simulink model "PROJECT_SIMULINK_LINEAR_BICYCLE_VLiam3"  (R2023b)
settings: Solver=ode4  StartTime=0.0  StopTime=20  FixedStep=1e-3  RelTol=1e-3  EnableMultiTasking=on
values from neighbouring files (symbols this model uses):
  Ts = 0.01    [PROJECT_INIT_LINEAR_BICYCLE_VLiam3.m]
  V_ref = 60 /3.6    (= 16.6666666667)    [PROJECT_INIT_LINEAR_BICYCLE_VLiam3.m]    (also in run_template.m)
undefined symbols (not defined in the file or in its folder): data, init, input, par
libraries: simulink x2
settings Model: Creator=bshyrokau  LastModifiedBy=liamr
settings SolverCC: AlgebraicLoopSolver=TrustRegion  AutoInsertRateTranBlk=on
settings DataIOCC: SaveOutput=off  SignalLogging=off  DSMLogging=off  SaveTime=off  ReturnWorkspaceOutputs=off
settings OptimizationCC: ReuseModelBlockBuffer=off  LifeSpan=inf
settings DebuggingCC: UnconnectedInputMsg=warning  UnconnectedOutputMsg=warning  UnconnectedLineMsg=warning  AllowSymbolicDim=off  SFUnexpectedBacktrackingDiag=warning  SFNoUnconditionalDefaultTransitionDiag=warning  SFExecutionAtInitializationDiag=none  ArithmeticOperatorsInVariantConditions=warning
settings ModelReferenceCC: EnableRefExpFcnMdlSchedulingChecks=on  PropagateSignalLabelsOutOfModel=off
settings SFSimCC: SimUseLocalCustomCode=off  CustomCodeUndefinedFunction=UseInterfaceOnly
settings RTWCC: RTWUseLocalCustomCode=off  DLArmComputeVersion=19.05
settings CodeAppCC: StateflowObjectComments=on
settings GRTTargetCC: TargetLangStandard=C89/C90 (ANSI)
settings ConfigComp: CovMetricSettings=dw  CovSaveCumulativeToWorkspaceVar=on  CovSaveSingleToWorkspaceVar=on  CovExternalEMLEnable=off
settings SimscapeCC: SimscapeNormalizeSystem=off
settings ConfigurationSet: Description=SimMechanics 2G

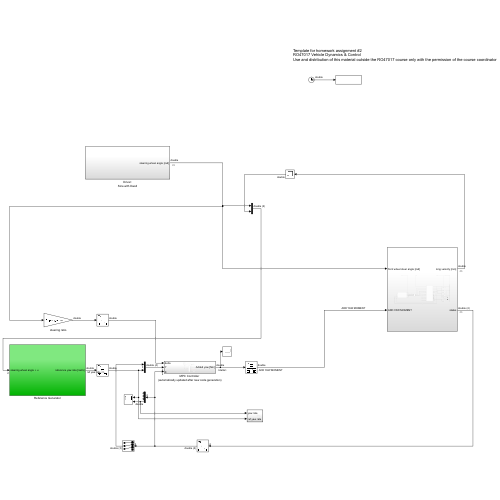
[thumbnail: Simulink's stored preview of the top-level diagram]
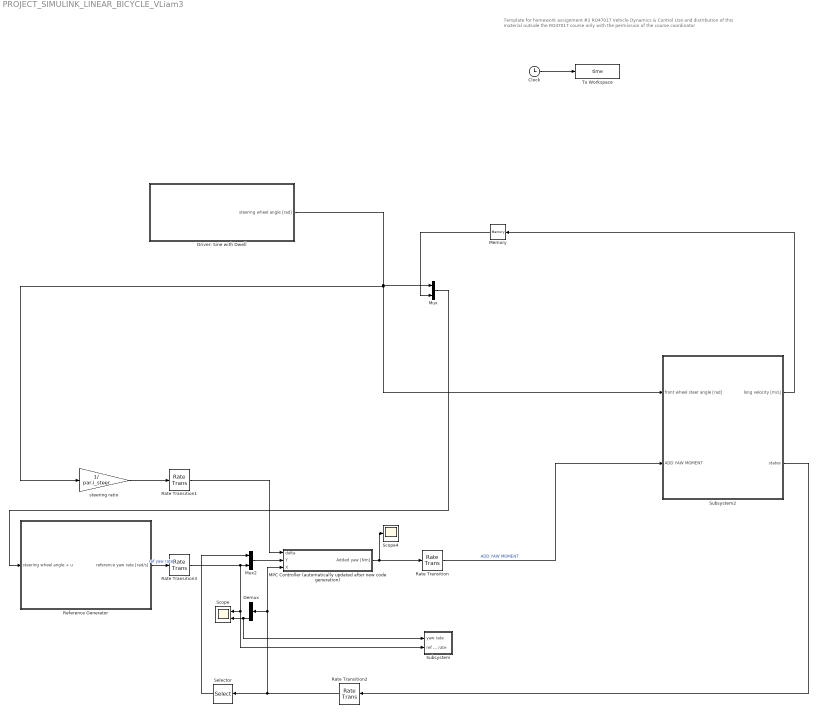
== system PROJECT_SIMULINK_LINEAR_BICYCLE_VLiam3 ==
  note: Template for homework assignment #2
      | RO47017 Vehicle Dynamics & Control
      | Use and distribution of this material outside the RO47017 course only with the permission of the course coordinator
  Clock : Clock
  Demux : Demux
  Driver: Sine with Dwell : Subsystem
  MPC Controller (automatically updated after new code generation) : Subsystem
  Memory : Memory
  Mux : Mux  Inputs=2
  Mux2 : Mux  Inputs=2
  Rate Transition : RateTransition
  Rate Transition1 : RateTransition  OutPortSampleTime=Ts
  Rate Transition2 : RateTransition  OutPortSampleTime=Ts
  Rate Transition3 : RateTransition  OutPortSampleTime=Ts
  Reference Generator : Subsystem  StartFcn=veh_parameters
  Scope : Scope  NumInputPorts=2
  Scope4 : Scope
  Selector : Selector  InputPortWidth=4  IndexOptions=Index vector (dialog)  Indices=[1 2 3]  OutputSizes=1
  Subsystem : Subsystem
  Subsystem2 : Subsystem
  To Workspace : ToWorkspace  VariableName=time  SampleTime=-1
  steering ratio : Gain  Gain=1/ par.i_steer
  wires:
  Driver: Sine with Dwell/1(steering wheel angle [rad]) -> Subsystem2/1(front wheel steer angle [rad]), steering ratio/1, Mux/1
  Clock/1 -> To Workspace/1
  MPC Controller (automatically updated after new code generation)/1(Added yaw [Nm]) -> Scope4/1, Rate Transition/1
  Rate Transition2/1 -> Selector/1, Demux/1, MPC Controller (automatically updated after new code generation)/3(X)
  Mux/1 -> Reference Generator/1(steering wheel angle + u)
  Rate Transition1/1 -> MPC Controller (automatically updated after new code generation)/1(delta)
  Memory/1 -> Mux/2
  Reference Generator/1(reference yaw rate [rad/s]) -> Rate Transition3/1  "ref yaw rate"
  Selector/1 -> Mux2/1
  Rate Transition3/1 -> Subsystem/2(ref yaw rate), Scope/1, Mux2/2
  Mux2/1 -> MPC Controller (automatically updated after new code generation)/2(Y)
  steering ratio/1 -> Rate Transition1/1
  Demux/4 -> Subsystem/1(yaw rate), Scope/2
  Rate Transition/1 -> Subsystem2/2(ADD YAW MOMENT)  "ADD YAW MOMENT"
  Subsystem2/1(long velocity [m/s]) -> Memory/1
  Subsystem2/2(states) -> Rate Transition2/1

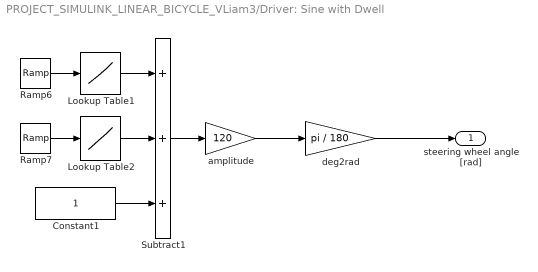
== system PROJECT_SIMULINK_LINEAR_BICYCLE_VLiam3/Driver: Sine with Dwell ==
  Constant1 : Constant
  Lookup Table1 : Lookup  InputValues=[0:0.1:3*pi/2 3*pi/2+eps]*0.7  Table=sin([0:0.1:3*pi/2 3*pi/2+eps])  LookUpMeth=Interpolation-Use End Values  SaturateOnIntegerOverflow=off
  Lookup Table2 : Lookup  InputValues=[3*pi/2:0.1:2*pi 2*pi+eps]*0.7  Table=sin([3*pi/2:0.1:2*pi 2*pi+eps])  LookUpMeth=Interpolation-Use End Values  SaturateOnIntegerOverflow=off
  Ramp6 : simulink/Sources/Ramp  slope=pi  start=10  InitialOutput=0
  Ramp7 : simulink/Sources/Ramp  slope=pi  start=10+0.5  InitialOutput=0
  Subtract1 : Sum  Inputs=+++
  amplitude : Gain  Gain=120
  deg2rad : Gain  Gain=pi / 180
  steering wheel angle [rad] : Outport  VectorParamsAs1DForOutWhenUnconnected=off
  wires:
  Ramp6/1 -> Lookup Table1/1
  Ramp7/1 -> Lookup Table2/1
  Lookup Table2/1 -> Subtract1/2
  Lookup Table1/1 -> Subtract1/1
  Constant1/1 -> Subtract1/3
  Subtract1/1 -> amplitude/1
  amplitude/1 -> deg2rad/1
  deg2rad/1 -> steering wheel angle [rad]/1

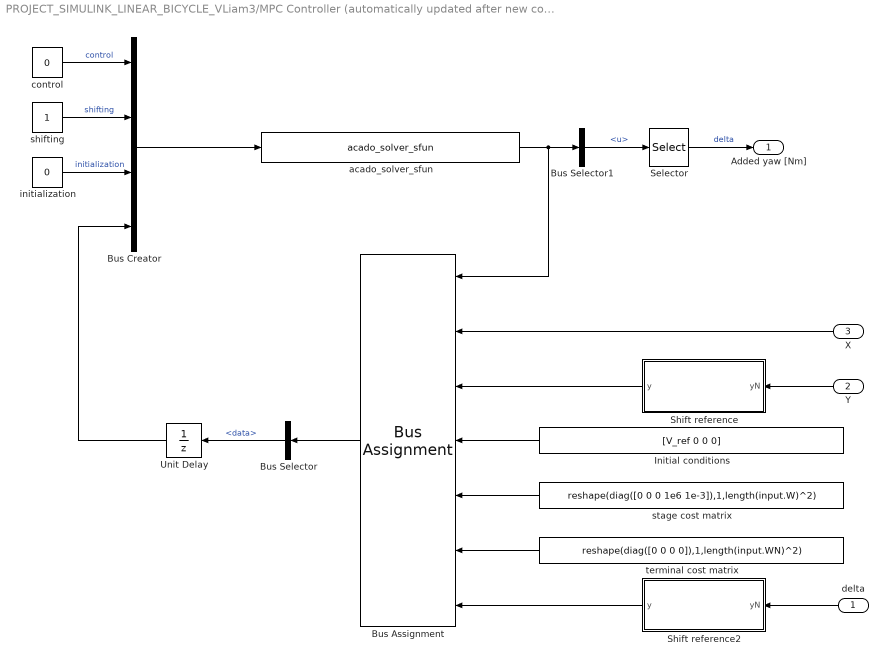
== system PROJECT_SIMULINK_LINEAR_BICYCLE_VLiam3/MPC Controller (automatically updated after new code generation) ==
  delta : Inport
  Y : Inport  Port=2
  X : Inport  Port=3
  Bus Assignment : BusAssignment  AssignedSignals=data.x0,data.y,data.yN,data.W,data.WN,data.od
  Bus Creator : BusCreator  Inputs=4  OutDataTypeStr=Bus: ACADOinput
  Bus Selector : BusSelector  OutputSignals=data
  Bus Selector1 : BusSelector  OutputSignals=data.u
  Initial conditions : Constant  Value=[V_ref 0 0 0]
  Selector : Selector  InputPortWidth=Np  IndexOptions=Starting index (dialog)  Indices=[1]  OutputSizes=1
  Shift reference : MATLAB Function  TreatAsAtomicUnit=on
  Shift reference2 : MATLAB Function  TreatAsAtomicUnit=on
  Unit Delay : UnitDelay  InitialCondition=init  SampleTime=Ts  HasFrameUpgradeWarning=on
  acado_solver_sfun : S-Function  FunctionName=acado_solver_sfun  SFunctionDeploymentMode=off  EnableBusSupport=off  mask(Legacy Function){SFunctionSpec=acado_step(ACADOinput u1[1], ACADOoutput y1[1]), ShowSpec=on}
      mask prompts: ShowSpec "Display function specification"
      mask help:
      | This block allows you to call the legacy functions specified by the following Legacy Code Tool definition:
      | def.SFunctionName = 'acado_solver_sfun';
      | def.OutputFcnSpec = 'acado_step(ACADOinput u1[1], ACADOoutput y1[1])';
      | def.StartFcnSpec = 'acado_initialize( void )';
      | def.TerminateFcnSpec = 'acado_cleanup( void )';
      | def.HeaderFiles = {'acado_common.h', 'acado_solver_sfunction.h'};
      | def.SourceFiles = {'acado_solver.c', 'acado_integrator.c', 'acado_auxiliary_functions.c', 'acado_solver_sfunction.c', 'acado_qpoases3_interface.c', 'qpoases3\src\Bounds.c', 'qpoases3\src\Constraints.c', 'qpoases3\src\Indexlist.c', 'qpoases3\src\Matrices.c', 'qpoases3\src\MessageHandling.c', 'qpoases3\src\Options.c', 'qpoases3\src\Flipper.c', 'qpoases3\src\QProblem.c', 'qpoases3\src\QProblemB.c', 'qpoases3\src\Utils.c'};
      mask Help: <p>This block was generated automatically by the Legacy Code Tool. For detailed help on this tool, call<a href="matlab:legacy_code('help')"> legacy_code('help')</a>.</p>
      mask Callback ShowSpec:
      | if strcmp(get_param(gcbh, 'ShowSpec'), 'on')
      |   set_param(gcbh, 'MaskDisplay', sprintf('fprintf(''%s'');', get_param(gcbh, 'SFunctionSpec')));
      | else
      |   set_param(gcbh, 'MaskDisplay', sprintf('fprintf(''%s'');', get_param(gcbh, 'FunctionName')));
      | end
      mask Display: fprintf('acado_step(ACADOinput u1[1], ACADOoutput y1[1])');
  control : Constant  Value=0  OutDataTypeStr=int32
  initialization : Constant  Value=0  OutDataTypeStr=int32
  shifting : Constant  OutDataTypeStr=int32
  stage cost matrix : Constant  Value=reshape(diag([0 0 0 1e6 1e-3]),1,length(input.W)^2)
  terminal cost matrix : Constant  Value=reshape(diag([0 0 0 0]),1,length(input.WN)^2)
  Added yaw [Nm] : Outport
  wires:
  control/1 -> Bus Creator/1  "control"
  Bus Selector1/1 -> Selector/1  "<u>"
  initialization/1 -> Bus Creator/3  "initialization"
  acado_solver_sfun/1 -> Bus Selector1/1, Bus Assignment/1
  shifting/1 -> Bus Creator/2  "shifting"
  Bus Assignment/1 -> Bus Selector/1
  terminal cost matrix/1 -> Bus Assignment/6
  Initial conditions/1 -> Bus Assignment/4
  Shift reference/1(y) -> Bus Assignment/3
  stage cost matrix/1 -> Bus Assignment/5
  Bus Selector/1 -> Unit Delay/1  "<data>"
  Unit Delay/1 -> Bus Creator/4
  Bus Creator/1 -> acado_solver_sfun/1
  Selector/1 -> Added yaw [Nm]/1  "delta"
  Y/1 -> Shift reference/1(yN)
  delta/1 -> Shift reference2/1(yN)
  X/1 -> Bus Assignment/2
  Shift reference2/1(y) -> Bus Assignment/7

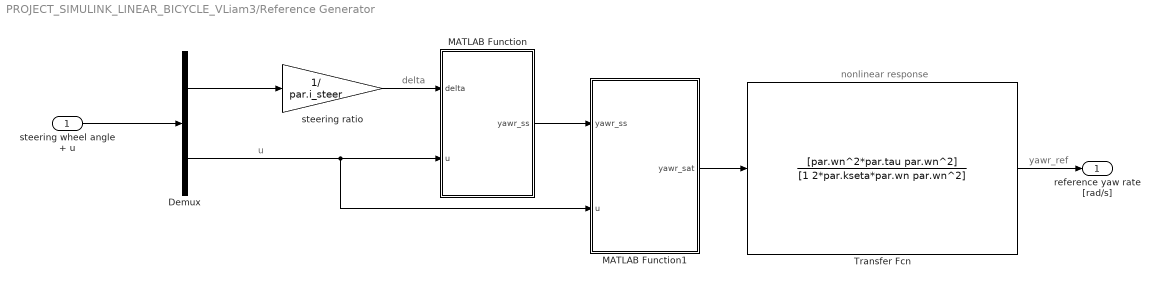
== system PROJECT_SIMULINK_LINEAR_BICYCLE_VLiam3/Reference Generator ==
  note: yawr_ref
  note: nonlinear response
  note: delta
  note: u
  steering wheel angle + u : Inport
  Demux : Demux  Outputs=2
  MATLAB Function : MATLAB Function  TreatAsAtomicUnit=on
  MATLAB Function1 : MATLAB Function  TreatAsAtomicUnit=on
  Transfer Fcn : TransferFcn  InitFcn=veh_parameters  StartFcn=veh_parameters  Numerator=[par.wn^2*par.tau par.wn^2]  Denominator=[1 2*par.kseta*par.wn par.wn^2]
  steering ratio : Gain  Gain=1/ par.i_steer
  reference yaw rate [rad/s] : Outport  VectorParamsAs1DForOutWhenUnconnected=off
  wires:
  steering ratio/1 -> MATLAB Function/1(delta)
  MATLAB Function/1(yawr_ss) -> MATLAB Function1/1(yawr_ss)
  MATLAB Function1/1(yawr_sat) -> Transfer Fcn/1
  Transfer Fcn/1 -> reference yaw rate [rad/s]/1
  Demux/1 -> steering ratio/1
  Demux/2 -> MATLAB Function1/2(u), MATLAB Function/2(u)
  steering wheel angle + u/1 -> Demux/1

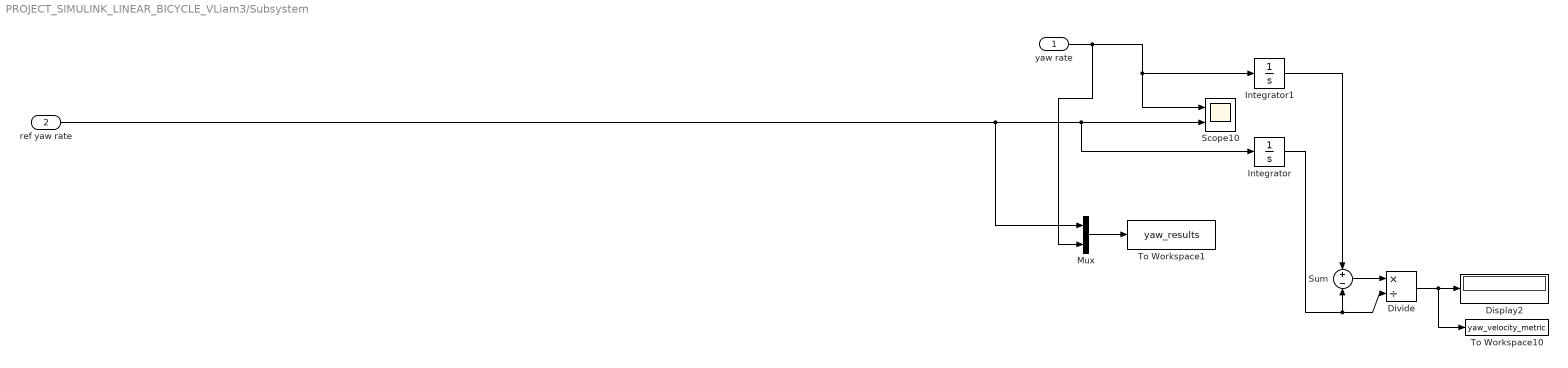
== system PROJECT_SIMULINK_LINEAR_BICYCLE_VLiam3/Subsystem ==
  yaw rate : Inport
  ref yaw rate : Inport  Port=2
  Display2 : Display
  Divide : Product  Inputs=*/
  Integrator : Integrator  InitialCondition=0.000001
  Integrator1 : Integrator
  Mux : Mux  Inputs=2
  Scope10 : Scope  NumInputPorts=2
  Sum : Sum  Inputs=+-
  To Workspace1 : ToWorkspace  VariableName=yaw_results  SaveFormat=Timeseries  SampleTime=-1
  To Workspace10 : ToWorkspace  VariableName=yaw_velocity_metric  SampleTime=-1
      settings: MaxDataPoints=1
  wires:
  yaw rate/1 -> Mux/2, Scope10/1, Integrator1/1
  ref yaw rate/1 -> Mux/1, Integrator/1, Scope10/2
  Divide/1 -> To Workspace10/1, Display2/1
  Integrator/1 -> Sum/2, Divide/2
  Integrator1/1 -> Sum/1
  Sum/1 -> Divide/1
  Mux/1 -> To Workspace1/1

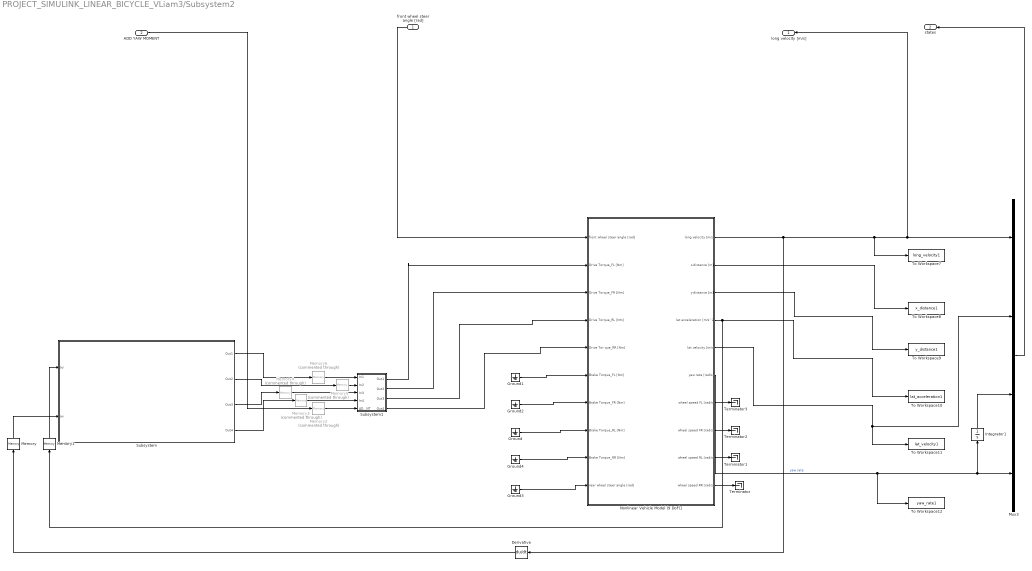
== system PROJECT_SIMULINK_LINEAR_BICYCLE_VLiam3/Subsystem2 ==
  front wheel steer angle [rad] : Inport
  ADD YAW MOMENT : Inport  Port=2
  Derivative : Derivative
  Ground{,1..4} (5 alike) : Ground
  Integrator1 : Integrator
  Memory : Memory
  Memory1 : Memory
  Memory{2..6} (5 alike) : Memory  Commented=through
  Mux3 : Mux
  Nonlinear Vehicle Model (9 DoF)1 : Subsystem
      mask help: Simulink:masks:GenSFuncDesc_MD
      mask Help: eval('feval(''rtwprivate'',''rtwhelpview'',''rtw_sfcn_block'')');
  Subsystem : Subsystem
  Subsystem1 : Subsystem
  Terminator{,1..3} (4 alike) : Terminator
  To Workspace10 : ToWorkspace  VariableName=lat_acceleration1  SampleTime=-1
  To Workspace11 : ToWorkspace  VariableName=lat_velocity1  SampleTime=-1
  To Workspace12 : ToWorkspace  VariableName=yaw_rate1  SampleTime=-1
  To Workspace7 : ToWorkspace  VariableName=long_velocity1  SampleTime=-1
  To Workspace8 : ToWorkspace  VariableName=x_distance1  SampleTime=-1
  To Workspace9 : ToWorkspace  VariableName=y_distance1  SampleTime=-1
  long velocity [m/s] : Outport
  states : Outport  Port=2
  wires:
  Subsystem1/1(Out1) -> Nonlinear Vehicle Model (9 DoF)1/2(Drive Torque_FL [Nm])
  Nonlinear Vehicle Model (9 DoF)1/1(long velocity [m/s]) -> Derivative/1, To Workspace7/1, long velocity [m/s]/1, Mux3/1
  Nonlinear Vehicle Model (9 DoF)1/4(lat acceleration [m/s^2]) -> To Workspace10/1, Memory1/1
  Nonlinear Vehicle Model (9 DoF)1/9(wheel speed RL [rad/s]) -> Terminator1/1
  Subsystem/3(Out3) -> Memory4/1
  Nonlinear Vehicle Model (9 DoF)1/6(yaw rate [rad/s]) -> Mux3/4, Integrator1/1, To Workspace12/1  "yaw rate"
  Ground/1 -> Nonlinear Vehicle Model (9 DoF)1/8(Brake Torque_RL [Nm])
  Nonlinear Vehicle Model (9 DoF)1/8(wheel speed FR [rad/s]) -> Terminator2/1
  Nonlinear Vehicle Model (9 DoF)1/2(x-distance [m]) -> To Workspace8/1
  Nonlinear Vehicle Model (9 DoF)1/3(y-distance [m]) -> To Workspace9/1
  Subsystem/1(Out1) -> Memory6/1
  Integrator1/1 -> Mux3/3
  Subsystem1/2(Out2) -> Nonlinear Vehicle Model (9 DoF)1/3(Drive Torque_FR [Nm])
  Nonlinear Vehicle Model (9 DoF)1/7(wheel speed FL [rad/s]) -> Terminator3/1
  Ground2/1 -> Nonlinear Vehicle Model (9 DoF)1/7(Brake Torque_FR [Nm])
  Subsystem/4(Out4) -> Memory3/1
  Subsystem1/3(Out3) -> Nonlinear Vehicle Model (9 DoF)1/4(Drive Torque_RL [Nm])
  Nonlinear Vehicle Model (9 DoF)1/5(lat velocity [m/s]) -> Mux3/2, To Workspace11/1
  Ground3/1 -> Nonlinear Vehicle Model (9 DoF)1/10(rear wheel steer angle [rad])
  Subsystem/2(Out2) -> Memory5/1
  Subsystem1/4(Out4) -> Nonlinear Vehicle Model (9 DoF)1/5(Drive Tor	que_RR [Nm])
  front wheel steer angle [rad]/1 -> Nonlinear Vehicle Model (9 DoF)1/1(front wheel steer angle [rad])
  Ground4/1 -> Nonlinear Vehicle Model (9 DoF)1/9(Brake Torque_RR [Nm])
  Ground1/1 -> Nonlinear Vehicle Model (9 DoF)1/6(Brake Torque_FL [Nm])
  Mux3/1 -> states/1
  Nonlinear Vehicle Model (9 DoF)1/10(wheel speed RR [rad/s]) -> Terminator/1
  ADD YAW MOMENT/1 -> Memory2/1
  Derivative/1 -> Memory/1
  Memory/1 -> Subsystem/2(ax)
  Memory1/1 -> Subsystem/1(ay)
  Memory2/1 -> Subsystem1/5(ADD YAW MOMENT)
  Memory3/1 -> Subsystem1/4(In4)
  Memory4/1 -> Subsystem1/3(In3)
  Memory5/1 -> Subsystem1/2(In2)
  Memory6/1 -> Subsystem1/1(In1)

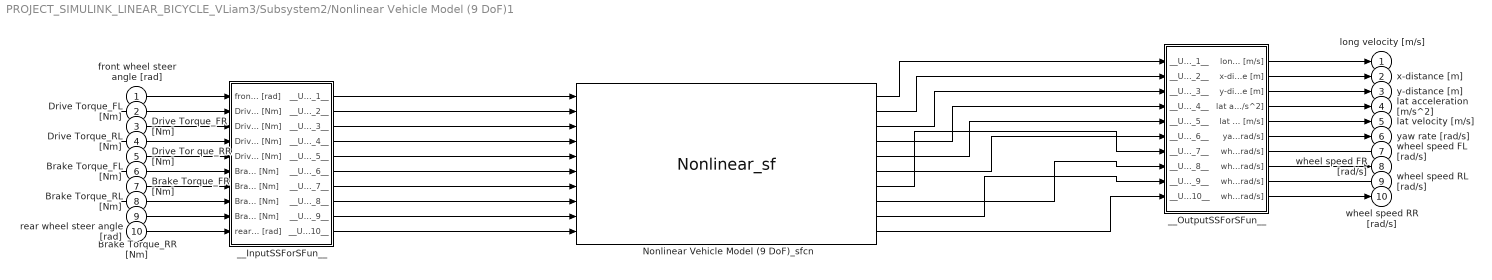
== system PROJECT_SIMULINK_LINEAR_BICYCLE_VLiam3/Subsystem2/Nonlinear Vehicle Model (9 DoF)1 ==
  front wheel steer angle [rad] : Inport
  Drive Torque_FL [Nm] : Inport  Port=2
  Drive Torque_FR [Nm] : Inport  Port=3
  Drive Torque_RL [Nm] : Inport  Port=4
  Drive Tor	que_RR [Nm] : Inport  Port=5
  Brake Torque_FL [Nm] : Inport  Port=6
  Brake Torque_FR [Nm] : Inport  Port=7
  Brake Torque_RL [Nm] : Inport  Port=8
  Brake Torque_RR [Nm] : Inport  Port=9
  rear wheel steer angle [rad] : Inport  Port=10
  Nonlinear Vehicle Model (9 DoF)_sfcn : S-Function  FunctionName=Nonlinear_sf  SFunctionModules=""  SFunctionDeploymentMode=off  EnableBusSupport=off  mask{rtw_sf_name=Nonlinear_sf, showVar=off}
      mask prompts: rtw_sf_name "Simulink:masks:GenSFuncName_MP"; showVar "Simulink:masks:GenSFuncShowModuleList_MP"
      mask help: Simulink:masks:GenSFuncDesc_MD
      mask init:
      | displist = '';
      | if ~strcmp(get_param(gcb, 'FunctionName'), rtw_sf_name);
      |   set_param(gcb, 'FunctionName', rtw_sf_name);
      | end
      | % Check if we are generating code
      | rtw_mode = false;
      | if strcmpi(get_param(bdroot(gcb),'SimulationStatus'),'Initializing')
      | 	rtw_mode = strcmpi(get_param(bdroot(gcb),'BuildingRTWCode'),'on') && ...
      | 		~strcmpi(get_param(bdroot(gcb),'TargetStyle'),'SimulationTarget');
      | end
      | if showVar || rtw_mode
      | 	if exist('rtwsfunc') == 2 | exist('rtwsfunc') == 6
      | 		tmplist = rtwsfunc(rtw_sf_name,gcb);
      | 		tmplist = DAStudio.message('Simulink:masks:GenSFuncListOfModules_IC', tmplist);
      | 	elseif showVar
      | 		tmplist1 = DAStudio.message('Simulink:masks:GenSFuncListOfModules_IC', '');
      |         tmplist2 = DAStudio.message('Simulink:masks:GenSFuncNotLicensed_IC');
      |         tmplist = [tmplist1 tmplist2];
      |  	end
      | end
      | if showVar
      |   displist = tmplist;
      | end
      settings: CopyFcn=|
      | if ~strcmp(get_param(gcb,'Linkstatus'),'none') && ...
      | ~strcmp(get_param(gcb,'Linkstatus'),'implicit')
      |   set_param(gcb,'LinkStatus','none');
      | end
      mask Help: eval('feval(''rtwprivate'',''rtwhelpview'',''rtw_sfcn_block'')');
      mask Display:
      | port_label('input',1,'front wheel steer angle [rad]');
      | port_label('input',2,'Drive Torque_FL [Nm]');
      | port_label('input',3,'Drive Torque_FR [Nm]');
      | port_label('input',4,'Drive Torque_RL [Nm]');
      | port_label('input',5,'Drive Tor	que_RR [Nm]');
      | port_label('input',6,'Brake Torque_FL [Nm]');
      | port_label('input',7,'Brake Torque_FR [Nm]');
      | port_label('input',8,'Brake Torque_RL [Nm]');
      | port_label('input',9,'Brake Torque_RR [Nm]');
      | port_label('input',10,'rear wheel steer angle [rad]');
      | port_label('output',1,'long velocity [m/s]');
      | port_label('output',2,'x-distance [m]');
      | port_label('output',3,'y-distance [m]');
      | port_label('output',4,'lat acceleration [m/s^2]');
      | port_label('output',5,'lat velocity [m/s]');
      | port_label('output',6,'yaw rate [rad/s]');
      | port_label('output',7,'wheel speed FL [rad/s]');
      | port_label('output',8,'wheel speed FR [rad/s]');
      | port_label('output',9,'wheel speed RL [rad/s]');
      | port_label('output',10,'wheel speed RR [rad/s]');
  __InputSSForSFun__ : Subsystem
  __OutputSSForSFun__ : Subsystem
  long velocity [m/s] : Outport  VectorParamsAs1DForOutWhenUnconnected=off
  x-distance [m] : Outport  Port=2  VectorParamsAs1DForOutWhenUnconnected=off
  y-distance [m] : Outport  Port=3  VectorParamsAs1DForOutWhenUnconnected=off
  lat acceleration [m/s^2] : Outport  Port=4  VectorParamsAs1DForOutWhenUnconnected=off
  lat velocity [m/s] : Outport  Port=5  VectorParamsAs1DForOutWhenUnconnected=off
  yaw rate [rad/s] : Outport  Port=6  VectorParamsAs1DForOutWhenUnconnected=off
  wheel speed FL [rad/s] : Outport  Port=7  VectorParamsAs1DForOutWhenUnconnected=off
  wheel speed FR [rad/s] : Outport  Port=8  VectorParamsAs1DForOutWhenUnconnected=off
  wheel speed RL [rad/s] : Outport  Port=9  VectorParamsAs1DForOutWhenUnconnected=off
  wheel speed RR [rad/s] : Outport  Port=10  VectorParamsAs1DForOutWhenUnconnected=off
  wires:
  front wheel steer angle [rad]/1 -> __InputSSForSFun__/1(front wheel steer angle [rad])
  Drive Torque_FL [Nm]/1 -> __InputSSForSFun__/2(Drive Torque_FL [Nm])
  Drive Torque_FR [Nm]/1 -> __InputSSForSFun__/3(Drive Torque_FR [Nm])
  Drive Torque_RL [Nm]/1 -> __InputSSForSFun__/4(Drive Torque_RL [Nm])
  Drive Tor	que_RR [Nm]/1 -> __InputSSForSFun__/5(Drive Tor	que_RR [Nm])
  Brake Torque_FL [Nm]/1 -> __InputSSForSFun__/6(Brake Torque_FL [Nm])
  Brake Torque_FR [Nm]/1 -> __InputSSForSFun__/7(Brake Torque_FR [Nm])
  Brake Torque_RL [Nm]/1 -> __InputSSForSFun__/8(Brake Torque_RL [Nm])
  Brake Torque_RR [Nm]/1 -> __InputSSForSFun__/9(Brake Torque_RR [Nm])
  rear wheel steer angle [rad]/1 -> __InputSSForSFun__/10(rear wheel steer angle [rad])
  __InputSSForSFun__/1(__UniqueOutportName__1__) -> Nonlinear Vehicle Model (9 DoF)_sfcn/1
  __InputSSForSFun__/2(__UniqueOutportName__2__) -> Nonlinear Vehicle Model (9 DoF)_sfcn/2
  __InputSSForSFun__/3(__UniqueOutportName__3__) -> Nonlinear Vehicle Model (9 DoF)_sfcn/3
  __InputSSForSFun__/4(__UniqueOutportName__4__) -> Nonlinear Vehicle Model (9 DoF)_sfcn/4
  __InputSSForSFun__/5(__UniqueOutportName__5__) -> Nonlinear Vehicle Model (9 DoF)_sfcn/5
  __InputSSForSFun__/6(__UniqueOutportName__6__) -> Nonlinear Vehicle Model (9 DoF)_sfcn/6
  __InputSSForSFun__/7(__UniqueOutportName__7__) -> Nonlinear Vehicle Model (9 DoF)_sfcn/7
  __InputSSForSFun__/8(__UniqueOutportName__8__) -> Nonlinear Vehicle Model (9 DoF)_sfcn/8
  __InputSSForSFun__/9(__UniqueOutportName__9__) -> Nonlinear Vehicle Model (9 DoF)_sfcn/9
  __InputSSForSFun__/10(__UniqueOutportName__10__) -> Nonlinear Vehicle Model (9 DoF)_sfcn/10
  Nonlinear Vehicle Model (9 DoF)_sfcn/1 -> __OutputSSForSFun__/1(__UniqueInportName__1__)
  Nonlinear Vehicle Model (9 DoF)_sfcn/2 -> __OutputSSForSFun__/2(__UniqueInportName__2__)
  Nonlinear Vehicle Model (9 DoF)_sfcn/3 -> __OutputSSForSFun__/3(__UniqueInportName__3__)
  Nonlinear Vehicle Model (9 DoF)_sfcn/4 -> __OutputSSForSFun__/4(__UniqueInportName__4__)
  Nonlinear Vehicle Model (9 DoF)_sfcn/5 -> __OutputSSForSFun__/5(__UniqueInportName__5__)
  Nonlinear Vehicle Model (9 DoF)_sfcn/6 -> __OutputSSForSFun__/6(__UniqueInportName__6__)
  Nonlinear Vehicle Model (9 DoF)_sfcn/7 -> __OutputSSForSFun__/7(__UniqueInportName__7__)
  Nonlinear Vehicle Model (9 DoF)_sfcn/8 -> __OutputSSForSFun__/8(__UniqueInportName__8__)
  Nonlinear Vehicle Model (9 DoF)_sfcn/9 -> __OutputSSForSFun__/9(__UniqueInportName__9__)
  Nonlinear Vehicle Model (9 DoF)_sfcn/10 -> __OutputSSForSFun__/10(__UniqueInportName__10__)
  __OutputSSForSFun__/1(long velocity [m/s]) -> long velocity [m/s]/1
  __OutputSSForSFun__/2(x-distance [m]) -> x-distance [m]/1
  __OutputSSForSFun__/3(y-distance [m]) -> y-distance [m]/1
  __OutputSSForSFun__/4(lat acceleration [m/s^2]) -> lat acceleration [m/s^2]/1
  __OutputSSForSFun__/5(lat velocity [m/s]) -> lat velocity [m/s]/1
  __OutputSSForSFun__/6(yaw rate [rad/s]) -> yaw rate [rad/s]/1
  __OutputSSForSFun__/7(wheel speed FL [rad/s]) -> wheel speed FL [rad/s]/1
  __OutputSSForSFun__/8(wheel speed FR [rad/s]) -> wheel speed FR [rad/s]/1
  __OutputSSForSFun__/9(wheel speed RL [rad/s]) -> wheel speed RL [rad/s]/1
  __OutputSSForSFun__/10(wheel speed RR [rad/s]) -> wheel speed RR [rad/s]/1

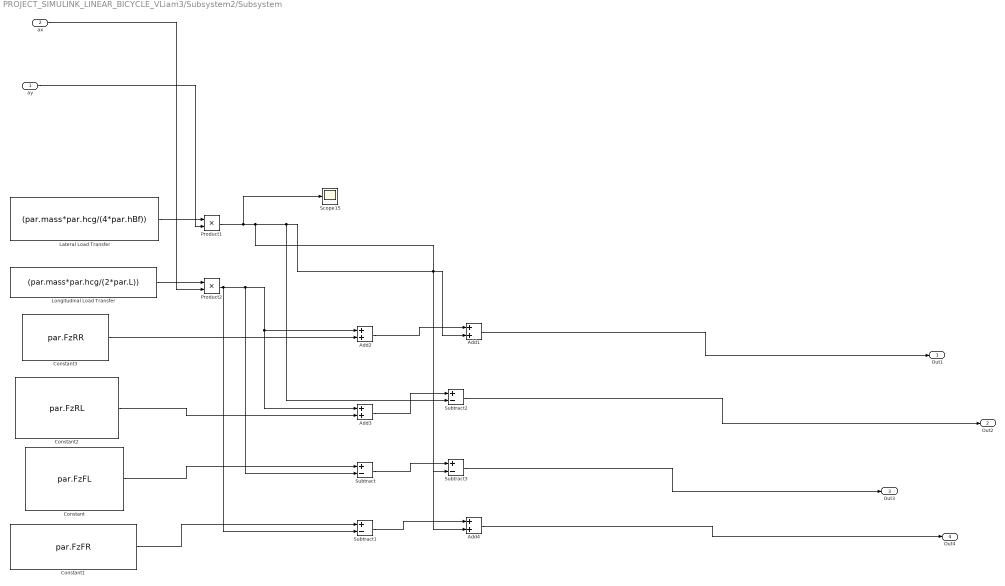
== system PROJECT_SIMULINK_LINEAR_BICYCLE_VLiam3/Subsystem2/Subsystem ==
  ay : Inport
  ax : Inport  Port=2
  Add{1..4} (4 alike) : Sum
  Constant : Constant  Value=par.FzFL
  Constant1 : Constant  Value=par.FzFR
  Constant2 : Constant  Value=par.FzRL
  Constant3 : Constant  Value=par.FzRR
  Lateral Load Transfer : Constant  Value=(par.mass*par.hcg/(4*par.hBf))
  Longitudinal Load Transfer : Constant  Value=(par.mass*par.hcg/(2*par.L))
  Product1 : Product
  Product2 : Product
  Scope15 : Scope
  Subtract{,1..3} (4 alike) : Sum  Inputs=+-
  Out1 : Outport
  Out2 : Outport  Port=2
  Out3 : Outport  Port=3
  Out4 : Outport  Port=4
  wires:
  Add4/1 -> Out4/1
  Add2/1 -> Add1/1
  Product1/1 -> Scope15/1, Add4/2, Subtract2/2, Subtract3/2, Add1/2
  Subtract/1 -> Subtract3/1
  Longitudinal Load Transfer/1 -> Product2/1
  Subtract1/1 -> Add4/1
  Product2/1 -> Subtract/2, Add3/1, Add2/1, Subtract1/2
  Add3/1 -> Subtract2/1
  Constant1/1 -> Subtract1/1
  Subtract3/1 -> Out3/1
  Constant2/1 -> Add3/2
  Lateral Load Transfer/1 -> Product1/1
  Constant3/1 -> Add2/2
  Subtract2/1 -> Out2/1
  Constant/1 -> Subtract/1
  ax/1 -> Product2/2
  Add1/1 -> Out1/1
  ay/1 -> Product1/2

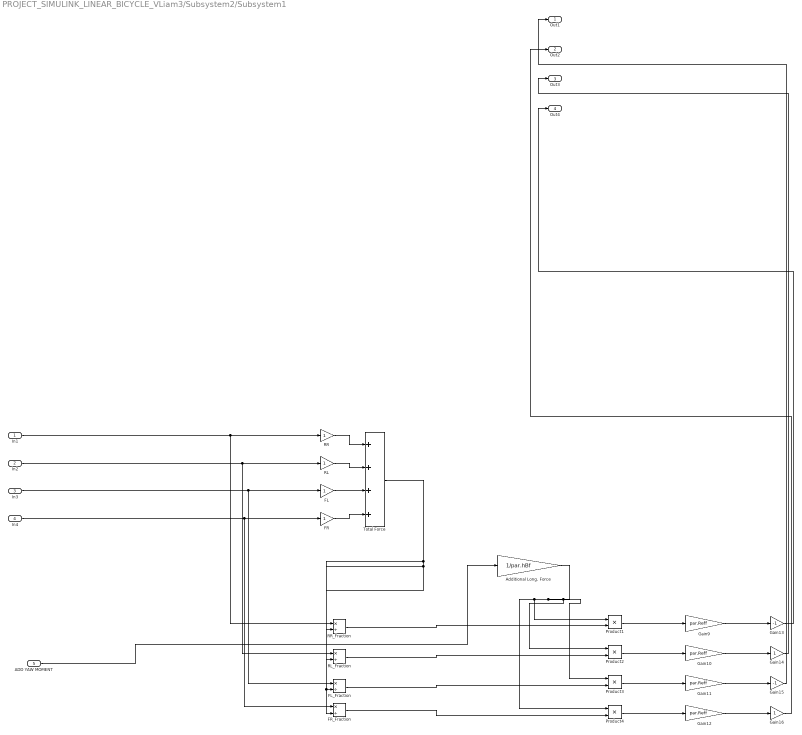
== system PROJECT_SIMULINK_LINEAR_BICYCLE_VLiam3/Subsystem2/Subsystem1 ==
  In1 : Inport
  In2 : Inport  Port=2
  In3 : Inport  Port=3
  In4 : Inport  Port=4
  ADD YAW MOMENT : Inport  Port=5
  Additional Long. Force : Gain  Gain=1/par.hBf
  FL : Gain
  FL_Fraction : Product  Inputs=*/
  FR : Gain
  FR_Fraction : Product  Inputs=*/
  Gain{9..12} (4 alike) : Gain  Gain=par.Reff
  Gain13 : Gain  Gain=-1
  Gain14 : Gain
  Gain15 : Gain  Gain=-1
  Gain16 : Gain
  Product{1..4} (4 alike) : Product
  RL : Gain
  RL_Fraction : Product  Inputs=*/
  RR : Gain
  RR_Fraction : Product  Inputs=*/
  Total Force : Sum  Inputs=++++
  Out1 : Outport
  Out2 : Outport  Port=2
  Out3 : Outport  Port=3
  Out4 : Outport  Port=4
  wires:
  RL/1 -> Total Force/2
  FR/1 -> Total Force/4
  In2/1 -> RL_Fraction/1, RL/1
  In3/1 -> FL/1, FL_Fraction/1
  Gain15/1 -> Out1/1
  Total Force/1 -> RL_Fraction/2, RR_Fraction/2, FL_Fraction/2, FR_Fraction/2
  Gain14/1 -> Out3/1
  Additional Long. Force/1 -> Product4/1, Product1/1, Product3/1, Product2/1
  FL/1 -> Total Force/3
  Product2/1 -> Gain10/1
  In4/1 -> FR_Fraction/1, FR/1
  In1/1 -> RR_Fraction/1, RR/1
  FL_Fraction/1 -> Product3/2
  Gain9/1 -> Gain13/1
  FR_Fraction/1 -> Product4/2
  RR_Fraction/1 -> Product1/2
  Gain12/1 -> Gain16/1
  RL_Fraction/1 -> Product2/2
  Product3/1 -> Gain11/1
  Product4/1 -> Gain12/1
  ADD YAW MOMENT/1 -> Additional Long. Force/1
  Product1/1 -> Gain9/1
  Gain10/1 -> Gain14/1
  Gain11/1 -> Gain15/1
  RR/1 -> Total Force/1
  Gain13/1 -> Out4/1
  Gain16/1 -> Out2/1

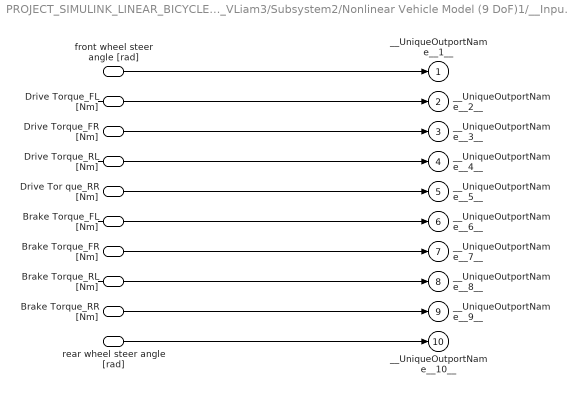
== system PROJECT_SIMULINK_LINEAR_BICYCLE_VLiam3/Subsystem2/Nonlinear Vehicle Model (9 DoF)1/__InputSSForSFun__ ==
  front wheel steer angle [rad] : Inport
  Drive Torque_FL [Nm] : Inport  Port=2
  Drive Torque_FR [Nm] : Inport  Port=3
  Drive Torque_RL [Nm] : Inport  Port=4
  Drive Tor	que_RR [Nm] : Inport  Port=5
  Brake Torque_FL [Nm] : Inport  Port=6
  Brake Torque_FR [Nm] : Inport  Port=7
  Brake Torque_RL [Nm] : Inport  Port=8
  Brake Torque_RR [Nm] : Inport  Port=9
  rear wheel steer angle [rad] : Inport  Port=10
  __UniqueOutportName__1__ : Outport
  __UniqueOutportName__2__ : Outport  Port=2
  __UniqueOutportName__3__ : Outport  Port=3
  __UniqueOutportName__4__ : Outport  Port=4
  __UniqueOutportName__5__ : Outport  Port=5
  __UniqueOutportName__6__ : Outport  Port=6
  __UniqueOutportName__7__ : Outport  Port=7
  __UniqueOutportName__8__ : Outport  Port=8
  __UniqueOutportName__9__ : Outport  Port=9
  __UniqueOutportName__10__ : Outport  Port=10
  wires:
  front wheel steer angle [rad]/1 -> __UniqueOutportName__1__/1
  Drive Torque_FL [Nm]/1 -> __UniqueOutportName__2__/1
  Drive Torque_FR [Nm]/1 -> __UniqueOutportName__3__/1
  Drive Torque_RL [Nm]/1 -> __UniqueOutportName__4__/1
  Drive Tor	que_RR [Nm]/1 -> __UniqueOutportName__5__/1
  Brake Torque_FL [Nm]/1 -> __UniqueOutportName__6__/1
  Brake Torque_FR [Nm]/1 -> __UniqueOutportName__7__/1
  Brake Torque_RL [Nm]/1 -> __UniqueOutportName__8__/1
  Brake Torque_RR [Nm]/1 -> __UniqueOutportName__9__/1
  rear wheel steer angle [rad]/1 -> __UniqueOutportName__10__/1

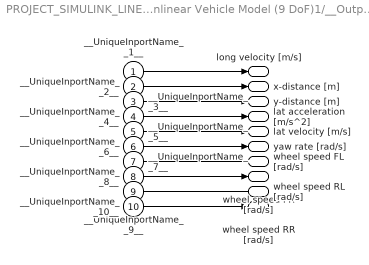
== system PROJECT_SIMULINK_LINEAR_BICYCLE_VLiam3/Subsystem2/Nonlinear Vehicle Model (9 DoF)1/__OutputSSForSFun__ ==
  __UniqueInportName__1__ : Inport
  __UniqueInportName__2__ : Inport  Port=2
  __UniqueInportName__3__ : Inport  Port=3
  __UniqueInportName__4__ : Inport  Port=4
  __UniqueInportName__5__ : Inport  Port=5
  __UniqueInportName__6__ : Inport  Port=6
  __UniqueInportName__7__ : Inport  Port=7
  __UniqueInportName__8__ : Inport  Port=8
  __UniqueInportName__9__ : Inport  Port=9
  __UniqueInportName__10__ : Inport  Port=10
  long velocity [m/s] : Outport  VectorParamsAs1DForOutWhenUnconnected=off
  x-distance [m] : Outport  Port=2  VectorParamsAs1DForOutWhenUnconnected=off
  y-distance [m] : Outport  Port=3  VectorParamsAs1DForOutWhenUnconnected=off
  lat acceleration [m/s^2] : Outport  Port=4  VectorParamsAs1DForOutWhenUnconnected=off
  lat velocity [m/s] : Outport  Port=5  VectorParamsAs1DForOutWhenUnconnected=off
  yaw rate [rad/s] : Outport  Port=6  VectorParamsAs1DForOutWhenUnconnected=off
  wheel speed FL [rad/s] : Outport  Port=7  VectorParamsAs1DForOutWhenUnconnected=off
  wheel speed FR [rad/s] : Outport  Port=8  VectorParamsAs1DForOutWhenUnconnected=off
  wheel speed RL [rad/s] : Outport  Port=9  VectorParamsAs1DForOutWhenUnconnected=off
  wheel speed RR [rad/s] : Outport  Port=10  VectorParamsAs1DForOutWhenUnconnected=off
  wires:
  __UniqueInportName__1__/1 -> long velocity [m/s]/1
  __UniqueInportName__2__/1 -> x-distance [m]/1
  __UniqueInportName__3__/1 -> y-distance [m]/1
  __UniqueInportName__4__/1 -> lat acceleration [m/s^2]/1
  __UniqueInportName__5__/1 -> lat velocity [m/s]/1
  __UniqueInportName__6__/1 -> yaw rate [rad/s]/1
  __UniqueInportName__7__/1 -> wheel speed FL [rad/s]/1
  __UniqueInportName__8__/1 -> wheel speed FR [rad/s]/1
  __UniqueInportName__9__/1 -> wheel speed RL [rad/s]/1
  __UniqueInportName__10__/1 -> wheel speed RR [rad/s]/1

== matlab function PROJECT_SIMULINK_LINEAR_BICYCLE_VLiam3/Reference Generator/MATLAB Function ==
  data: delta input; u input; yawr_ss output; par parameter
function yawr_ss = bicycle_model(delta,u,par)
%Parameters
L = par.L;
g = par.g;
m = par.mass;
K = par.Kus;

%Yaw rate response
yawr_ss = u*delta/(L+K*u^2/g);

== matlab function PROJECT_SIMULINK_LINEAR_BICYCLE_VLiam3/MPC Controller (automatically updated after new code generation)/Shift reference ==
  data: y output; yN input; Np parameter
function y = shift_reference(yN,Np)

y=repmat([yN;0],Np,1)';

end

== matlab function PROJECT_SIMULINK_LINEAR_BICYCLE_VLiam3/MPC Controller (automatically updated after new code generation)/Shift reference2 ==
  data: y output; yN input; Np parameter
function y = shift_reference(yN,Np)

y=repmat(yN,Np+1,1)';

end

== matlab function PROJECT_SIMULINK_LINEAR_BICYCLE_VLiam3/Reference Generator/MATLAB Function1 ==
  data: yawr_ss input; u input; yawr_sat output; par parameter
function yawr_sat = boundary_conditions(yawr_ss,u,par)
g = par.g;
mu = par.mu;

yawr_max = 0.85*mu*g/u;

if abs(yawr_ss) > abs(yawr_max)
    yawr_sat = sign(yawr_ss)*yawr_max;
else
    yawr_sat = yawr_ss;
end
